simulink model "Circuit_Overall"  (R2022a)
settings: Solver=VariableStepAuto  StartTime=0.0  StopTime=10.0  RelTol=1e-3
model workspace (MAT data in the model file):
  A_CT = [0  1  0  0; -0.3  -2  0.15  0; 0  0  0  1; 0.15  0  -0.15  0]
  A_ROM = [0.942562583619  0.116457352221  -0.0014011353287; -0.116491412917  -0.0147763560777  -0.0178750743564; -0.00153873683403  0.0687957046907  1.00005420683]
  A_est = [0.942562583619  0.116457352221  -0.0014011353287; -0.116491412917  -0.0147763560777  -0.0178750743564; -0.00153873683403  0.0687957046907  1.00005420683]
  B_CT = [0; 0.2; 0; 0]
  B_ROM = [-0.212642537526; -0.212676541741; -0.000489555407657]
  B_est = [-0.212642537526; -0.212676541741; -0.000489555407657]
  C = [0 0 1]
  C1 = 1e-06
  C4 = 0.0001
  C_ROM = [-0.000607137408501 0.00058416126542 0.00993914029103]
  C_est = [-0.000607137408501 0.00058416126542 0.00993914029103]
  F_in = 1
  Iden = [1  0  0; 0  1  0; 0  0  1]
  InputSignal = [0 5.00500500501e-08 1.001001001e-07 1.5015015015e-07 2.002002002e-07 2.5025025025e-07 3.003003003e-07 3.5035035035e-07 4.004004004e-07 4.5045045045e-07 5.00500500501e-07 5.50550550551e-07 ... (2000 elements, 1000x2)]
  K_infty = [-0.0307353179564; 0.00185109106169; 0.108053615593]
  P_k_0 = [0.5  0  0; 0  0.5  0; 0  0  0.5]
  Q = 0.1
  R = 0.001
  R1 = 2
  R2 = 2
  R3 = 2
  R4 = 2
  Ts = 1e-07
  Vs = 1
  b = 10
  k1 = 0.75
  k2 = 0.75
  m1 = 5
  m2 = 5
  omega = 3141592.65359
  x0 = [0; 0; 0; 0]
  x0_2D = [0; 0]
  x0_ROM = [0; 0; 0]
  x0_est = [0; 0; 0]
  x_0_est = [0; 0; 0; 0]
settings Model: Creator=tyevans  LastModifiedBy=tyevans

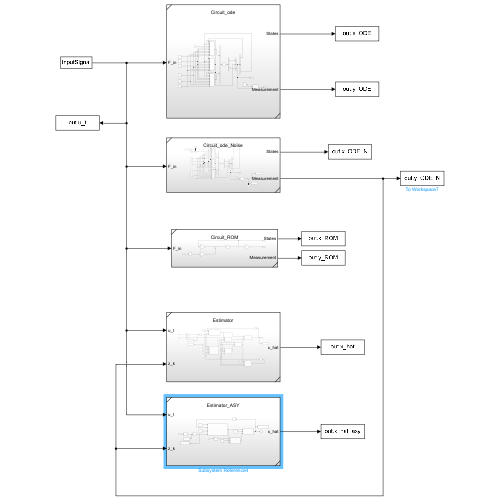
[thumbnail: Simulink's stored preview of the top-level diagram]
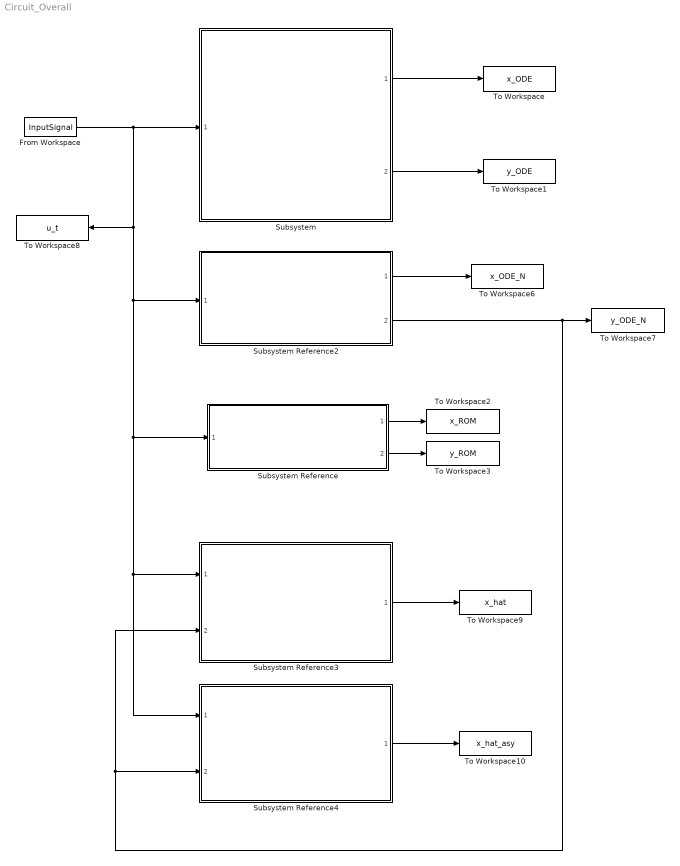
== system Circuit_Overall ==
  From Workspace : FromWorkspace  VariableName=InputSignal  OutputAfterFinalValue=Setting to zero
  Subsystem : Subsystem  ReferencedSubsystem=Circuit_ode
  Subsystem Reference : Subsystem  ReferencedSubsystem=Circuit_ROM
  Subsystem Reference2 : Subsystem  ReferencedSubsystem=Circuit_ode_Noise
  Subsystem Reference3 : Subsystem  ReferencedSubsystem=Estimator
  Subsystem Reference4 : Subsystem  ReferencedSubsystem=Estimator_ASY
  To Workspace : ToWorkspace  VariableName=x_ODE  SaveFormat=Structure With Time  SampleTime=-1
  To Workspace1 : ToWorkspace  VariableName=y_ODE  SaveFormat=Structure With Time  SampleTime=-1
  To Workspace10 : ToWorkspace  VariableName=x_hat_asy  SaveFormat=Structure With Time  SampleTime=-1
  To Workspace2 : ToWorkspace  VariableName=x_ROM  SaveFormat=Structure With Time  SampleTime=-1
  To Workspace3 : ToWorkspace  VariableName=y_ROM  SaveFormat=Structure With Time  SampleTime=-1
  To Workspace6 : ToWorkspace  VariableName=x_ODE_N  SaveFormat=Structure With Time  SampleTime=-1
  To Workspace7 : ToWorkspace  VariableName=y_ODE_N  SaveFormat=Structure With Time  SampleTime=-1
  To Workspace8 : ToWorkspace  VariableName=u_t  SaveFormat=Structure With Time  SampleTime=-1
  To Workspace9 : ToWorkspace  VariableName=x_hat  SaveFormat=Structure With Time  SampleTime=-1
  wires:
  Subsystem/1 -> To Workspace/1
  Subsystem/2 -> To Workspace1/1
  Subsystem Reference2/1 -> To Workspace6/1
  Subsystem Reference3/1 -> To Workspace9/1
  From Workspace/1 -> To Workspace8/1, Subsystem Reference/1, Subsystem Reference4/1, Subsystem Reference3/1, Subsystem Reference2/1, Subsystem/1
  Subsystem Reference2/2 -> Subsystem Reference4/2, Subsystem Reference3/2, To Workspace7/1
  Subsystem Reference4/1 -> To Workspace10/1
  Subsystem Reference/1 -> To Workspace2/1
  Subsystem Reference/2 -> To Workspace3/1
